simulink model "EE_Lab3"  (R2024b)
settings: Solver=VariableStepAuto  StartTime=0.0  StopTime=.04  RelTol=1e-3
libraries: spsRMSLib x7, eePowerMeasurement x4, spsVoltageMeasurementLib x4, spsSeriesRLCLoadLib x3, spsCurrentMeasurementLib x3, spsACVoltageSourceLib x2, spsGroundLib x2, spsSeriesRLCBranchLib x2, spspowerguiLib x2
settings Model: Creator=offic  LastModifiedBy=offic

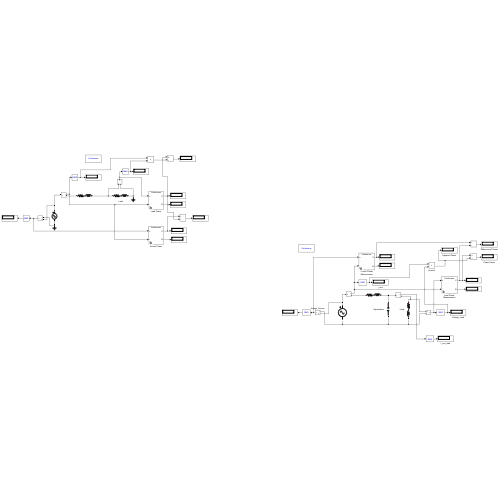
[thumbnail: Simulink's stored preview of the top-level diagram]
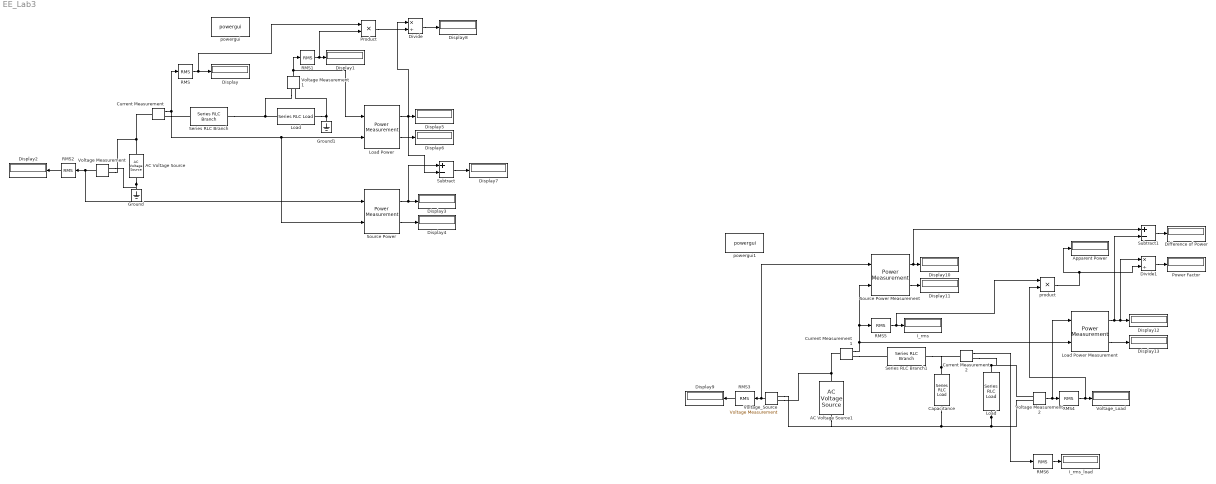
== system EE_Lab3 ==
  " Load" : spsSeriesRLCLoadLib/Series RLC Load  LConnTagsString=a  RConnTagsString=__new0  NominalVoltage=155.6  NominalFrequency=50  ActivePower=100  InductivePower=90  CapacitivePower=0  Setx0=off  InitialVoltage=0  SetiL0=off  InitialCurrent=0  Measurements=None  LoadType=constant Z
  AC Voltage Source : spsACVoltageSourceLib/AC Voltage Source  Amplitude=220  Phase=0  Frequency=50  SampleTime=0  Measurements=None  BusType=swing  Pref=10e3  Qref=0  Qmin=-inf  Qmax=+inf
  AC Voltage Source1 : spsACVoltageSourceLib/AC Voltage Source  Amplitude=220  Phase=0  Frequency=50  SampleTime=0  Measurements=None  BusType=swing  Pref=10e3  Qref=0  Qmin=-inf  Qmax=+inf
  Apparent Power : Display
  Capacitance : spsSeriesRLCLoadLib/Series RLC Load  LConnTagsString=a  RConnTagsString=__new0  NominalVoltage=155.6  NominalFrequency=50  ActivePower=0  InductivePower=0  CapacitivePower=90  Setx0=off  InitialVoltage=0  SetiL0=off  InitialCurrent=0  Measurements=None  LoadType=constant Z
  Current Measurement : spsCurrentMeasurementLib/Current Measurement  PhasorSimulation=off  OutputType=Complex  PSBequivalent=0
  Current Measurement1 : spsCurrentMeasurementLib/Current Measurement  PhasorSimulation=off  OutputType=Complex  PSBequivalent=0
  Current Measurement2 : spsCurrentMeasurementLib/Current Measurement  PhasorSimulation=off  OutputType=Complex  PSBequivalent=0
  Difference of Power : Display
  Display{,1..13} (14 alike) : Display
  Divide : Product  Inputs=*/
  Divide1 : Product  Inputs=*/
  Ground : spsGroundLib/Ground  LConnTagsString=a
  Ground1 : spsGroundLib/Ground  LConnTagsString=a
  I_rms : Display
  I_rms_load : Display
  Load : spsSeriesRLCLoadLib/Series RLC Load  LConnTagsString=a  RConnTagsString=__new0  NominalVoltage=155.6  NominalFrequency=50  ActivePower=100  InductivePower=90  CapacitivePower=0  Setx0=off  InitialVoltage=0  SetiL0=off  InitialCurrent=0  Measurements=None  LoadType=constant Z
  Load Power : eePowerMeasurement/Power Measurement  LabelModeActiveChoice=Continuous  F=50  K=[1]  Ts=0
  Load Power Measurement : eePowerMeasurement/Power Measurement  LabelModeActiveChoice=Continuous  F=50  K=[1]  Ts=0
  Power Factor : Display
  Product : Product
  RMS{,1..6} (7 alike) : spsRMSLib/RMS  TrueRMS=on  Freq=50  RMSInit=120  Ts=0
  Series RLC Branch : spsSeriesRLCBranchLib/Series RLC Branch  LConnTagsString=__new0  RConnTagsString=__new0  BranchType=RL  Resistance=10  Inductance=1e-2  SetiL0=off  InitialCurrent=0  Capacitance=1e-6  Setx0=off  InitialVoltage=0  Measurements=None
  Series RLC Branch1 : spsSeriesRLCBranchLib/Series RLC Branch  LConnTagsString=__new0  RConnTagsString=__new0  BranchType=RL  Resistance=1  Inductance=0.001  SetiL0=off  InitialCurrent=0  Capacitance=1e-6  Setx0=off  InitialVoltage=0  Measurements=None
  Source Power : eePowerMeasurement/Power Measurement  LabelModeActiveChoice=Continuous  F=50  K=[1]  Ts=0
  Source Power Measurement : eePowerMeasurement/Power Measurement  LabelModeActiveChoice=Continuous  F=50  K=[1]  Ts=0
  Subtract : Sum  Inputs=+-
  Subtract1 : Sum  Inputs=+-
  Voltage Measurement : spsVoltageMeasurementLib/Voltage Measurement  PhasorSimulation=off  OutputType=Complex  PSBequivalent=0
  Voltage Measurement1 : spsVoltageMeasurementLib/Voltage Measurement  PhasorSimulation=off  OutputType=Complex  PSBequivalent=0
  Voltage Measurement2 : spsVoltageMeasurementLib/Voltage Measurement  PhasorSimulation=off  OutputType=Complex  PSBequivalent=0
  Voltage_Load : Display
  Voltage_Source : spsVoltageMeasurementLib/Voltage Measurement  PhasorSimulation=off  OutputType=Complex  PSBequivalent=0
  powergui : spspowerguiLib/powergui  Priority=1  SimulationMode=Continuous  SampleTime=50e-6  frequency=60  Iterations=50  frequencyindice=50  Pbase=100e6  ErrMax=1e-4  UnitsV=kV  UnitsW=MW  buscounter=0  FunctionMessages=off  echomessages=off  EnableUseOfTLC=off  CurrentSourceSwitches=off  DisableSnubberDevices=off  DisableRonSwitches=off  DisableVfSwitches=off  DisplayEquations=off  AutomaticDiscreteSolvers=off  SolverType=Tustin/Backward Euler (TBE)  Interpol=off  ExternalGateDelay=off  methode=off  Ts=100  x0status=blocks  SPID=on  SwTol=0  HookPort=off  NonlinearTolerance=1e-4  nMaxIteration=100  ContinueOnMaxIteration=off  RestoreLinks=warning  ResistiveCurrentMeasurement=off  Frange=[0:2:500]  Ylog=off  Xlog=on  ShowGrid=off  save=off  variable=ZData  structure=0  ZoomFFT=off  StartTime=0.0  cycles=1  DisplayStyle=1  fundamental=60  FreqAxis=off  MaxFrequency=1000  frequencyindicesteady=1  RmsSteady=1  display=off
  powergui1 : spspowerguiLib/powergui  Priority=1  SimulationMode=Continuous  SampleTime=50e-6  frequency=60  Iterations=50  frequencyindice=50  Pbase=100e6  ErrMax=1e-4  UnitsV=kV  UnitsW=MW  buscounter=0  FunctionMessages=off  echomessages=off  EnableUseOfTLC=off  CurrentSourceSwitches=off  DisableSnubberDevices=off  DisableRonSwitches=off  DisableVfSwitches=off  DisplayEquations=off  AutomaticDiscreteSolvers=off  SolverType=Tustin/Backward Euler (TBE)  Interpol=off  ExternalGateDelay=off  methode=off  Ts=100  x0status=blocks  SPID=on  SwTol=0  HookPort=off  NonlinearTolerance=1e-4  nMaxIteration=100  ContinueOnMaxIteration=off  RestoreLinks=warning  ResistiveCurrentMeasurement=off  Frange=[0:2:500]  Ylog=off  Xlog=on  ShowGrid=off  save=off  variable=ZData  structure=0  ZoomFFT=off  StartTime=0.0  cycles=1  DisplayStyle=1  fundamental=60  FreqAxis=off  MaxFrequency=1000  frequencyindicesteady=1  RmsSteady=1  display=off
  product : Product
  wires:
  RMS/1 -> Product/1, Display/1
  Current Measurement/1 -> Load Power/2, Source Power/2, RMS/1
  RMS1/1 -> Product/2, Display1/1
  RMS2/1 -> Display2/1
  Voltage Measurement/1 -> RMS2/1, Source Power/1
  Voltage Measurement1/1 -> RMS1/1, Load Power/1
  Source Power/1 -> Subtract/1, Display3/1
  Source Power/2 -> Display4/1
  Load Power/2 -> Display6/1
  Load Power/1 -> Subtract/2, Divide/1, Display5/1
  Subtract/1 -> Display7/1
  Product/1 -> Divide/2
  Divide/1 -> Display8/1
  RMS5/1 -> product/1, I_rms/1
  Source Power Measurement/2 -> Display11/1
  RMS4/1 -> product/2, Voltage_Load/1
  Divide1/1 -> Power Factor/1
  Current Measurement2/1 -> RMS6/1
  Voltage Measurement2/1 -> Load Power Measurement/1, RMS4/1
  RMS6/1 -> I_rms_load/1
  Subtract1/1 -> Difference of Power/1
  Source Power Measurement/1 -> Subtract1/1, Display10/1
  RMS3/1 -> Display9/1
  Voltage_Source/1 -> Source Power Measurement/1, RMS3/1
  product/1 -> Divide1/2, Apparent Power/1
  Load Power Measurement/1 -> Subtract1/2, Divide1/1, Display12/1
  Load Power Measurement/2 -> Display13/1
  Current Measurement1/1 -> Load Power Measurement/2, RMS5/1, Source Power Measurement/2
  connections:
  Series RLC Branch/RConn1 -- Voltage Measurement1/LConn1 -- " Load"/LConn1
  Current Measurement/RConn1 -- Series RLC Branch/LConn1
  Current Measurement/LConn1 -- AC Voltage Source/RConn1 -- Voltage Measurement/LConn1
  Voltage Measurement/LConn2 -- Ground/LConn1 -- AC Voltage Source/LConn1
  " Load"/RConn1 -- Ground1/LConn1 -- Voltage Measurement1/LConn2
  Voltage_Source/LConn1 -- AC Voltage Source1/RConn1 -- Current Measurement1/LConn1
  Capacitance/LConn1 -- Series RLC Branch1/RConn1 -- Current Measurement2/LConn1
  Load/RConn1 -- Voltage Measurement2/LConn2 -- AC Voltage Source1/LConn1 -- Voltage_Source/LConn2 -- Capacitance/RConn1
  Load/LConn1 -- Voltage Measurement2/LConn1 -- Current Measurement2/RConn1
  Current Measurement1/RConn1 -- Series RLC Branch1/LConn1
